simulink model "vil_ut"  (Simulink 8.1)
settings: Solver=FixedStepDiscrete  StartTime=0.0  StopTime=10.0  FixedStep=0.005  RelTol=1e-3
libraries: siltestlib x11, idiada_lib x3, vil x1
settings Model: Creator=xsellart  LastModifiedBy=AT015555
settings DataIOCC: SignalLoggingSaveFormat=Dataset
settings OptimizationCC: ExpressionDepthLimit=128
settings DebuggingCC: FcnCallInpInsideContextMsg=EnableAllAsError
settings GRTTargetCC: CombineOutputUpdateFcns=on  GRTInterface=off

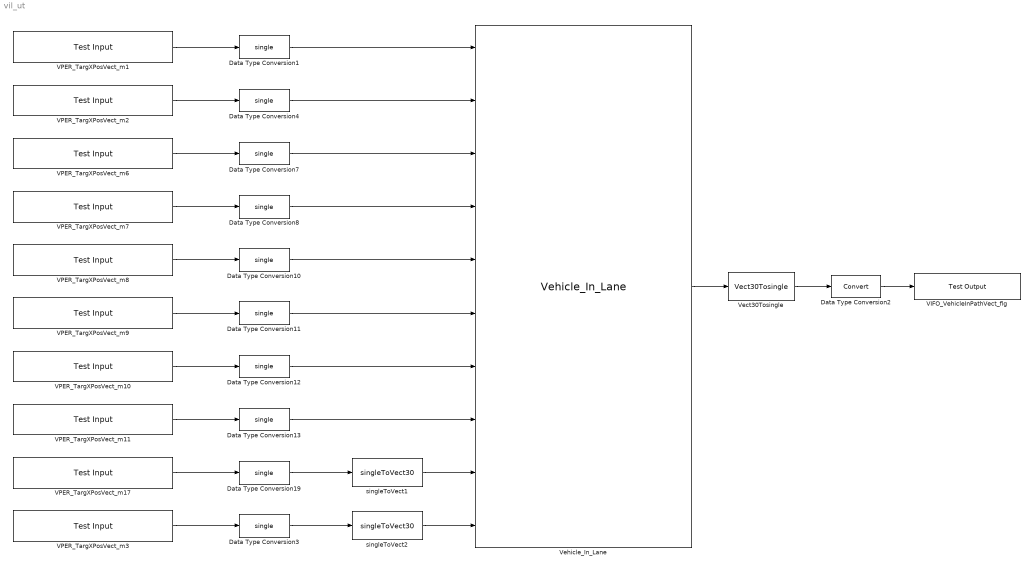
== system vil_ut ==
  Data Type Conversion{1,3..4,7..8,10..13,19} (10 alike) : DataTypeConversion  OutDataTypeStr=single
  Data Type Conversion2 : DataTypeConversion
  VIFO_VehicleInPathVect_flg : siltestlib/Test Output  varname=VIFO_TargetInLane_flg  sampletime=-1
  VPER_TargXPosVect_m1 : siltestlib/Test Input  varname=VPER_LaneC0L_m  sampletime=0.005
  VPER_TargXPosVect_m10 : siltestlib/Test Input  varname=VPER_LaneC2R_rat  sampletime=0.005
  VPER_TargXPosVect_m11 : siltestlib/Test Input  varname=VPER_LaneC3R_rat  sampletime=0.005
  VPER_TargXPosVect_m17 : siltestlib/Test Input  varname=VPER_TargXPosVect30_m  sampletime=0.005
  VPER_TargXPosVect_m2 : siltestlib/Test Input  varname=VPER_LaneC1L_rad  sampletime=0.005
  VPER_TargXPosVect_m3 : siltestlib/Test Input  varname=VPER_TargYPosVect30_m  sampletime=0.005
  VPER_TargXPosVect_m6 : siltestlib/Test Input  varname=VPER_LaneC2L_rat  sampletime=0.005
  VPER_TargXPosVect_m7 : siltestlib/Test Input  varname=VPER_LaneC3L_rat  sampletime=0.005
  VPER_TargXPosVect_m8 : siltestlib/Test Input  varname=VPER_LaneC0R_m  sampletime=0.005
  VPER_TargXPosVect_m9 : siltestlib/Test Input  varname=VPER_LaneC1R_rad  sampletime=0.005
  Vect30Tosingle : idiada_lib/Vect30Tosingle
  Vehicle_In_Lane : vil/Vehicle_In_Lane
  singleToVect1 : idiada_lib/singleToVect30
  singleToVect2 : idiada_lib/singleToVect30
  wires:
  Vect30Tosingle/1 -> Data Type Conversion2/1
  Data Type Conversion2/1 -> VIFO_VehicleInPathVect_flg/1
  Vehicle_In_Lane/1 -> Vect30Tosingle/1
  VPER_TargXPosVect_m1/1 -> Data Type Conversion1/1
  VPER_TargXPosVect_m2/1 -> Data Type Conversion4/1
  VPER_TargXPosVect_m6/1 -> Data Type Conversion7/1
  VPER_TargXPosVect_m7/1 -> Data Type Conversion8/1
  VPER_TargXPosVect_m8/1 -> Data Type Conversion10/1
  VPER_TargXPosVect_m9/1 -> Data Type Conversion11/1
  VPER_TargXPosVect_m10/1 -> Data Type Conversion12/1
  VPER_TargXPosVect_m11/1 -> Data Type Conversion13/1
  Data Type Conversion4/1 -> Vehicle_In_Lane/2
  Data Type Conversion13/1 -> Vehicle_In_Lane/8
  Data Type Conversion1/1 -> Vehicle_In_Lane/1
  Data Type Conversion8/1 -> Vehicle_In_Lane/4
  Data Type Conversion7/1 -> Vehicle_In_Lane/3
  Data Type Conversion12/1 -> Vehicle_In_Lane/7
  Data Type Conversion11/1 -> Vehicle_In_Lane/6
  Data Type Conversion10/1 -> Vehicle_In_Lane/5
  VPER_TargXPosVect_m17/1 -> Data Type Conversion19/1
  Data Type Conversion19/1 -> singleToVect1/1
  VPER_TargXPosVect_m3/1 -> Data Type Conversion3/1
  Data Type Conversion3/1 -> singleToVect2/1
  singleToVect1/1 -> Vehicle_In_Lane/9
  singleToVect2/1 -> Vehicle_In_Lane/10
